simulink model "model03"  (R2018b)
settings: Solver=FixedStepAuto  StartTime=0.0  StopTime=6  FixedStep=0.001  RelTol=1e-3
values from neighbouring files (symbols this model uses):
  A_sys = [0    1 ... (first row only)    [main.m]
  B_sys = [b1 ... (first row only)    [main.m]
  C_sys = eye(2)    [main.m]
  D_sys = [0 ... (first row only)    [main.m]
  gamma = 0.1    [data.m]
  init = [1 0; -b1*k 1]^-1 * init_conds(3,:)'    [main.m]
  k = 5    [main.m]
  k1 = b^2/((V^2*sin(lambda)-b*g*cos(lambda))*m*a*c*sin(lambda))    [main.m]    (also in plotRlocus.m = 0.06)
  k2 = b*g/(V^2*sin(lambda)-b*g*cos(lambda))    [main.m]    (also in plotRlocus.m = 1.95)
settings Model: Creator=franc  LastModifiedBy=franc

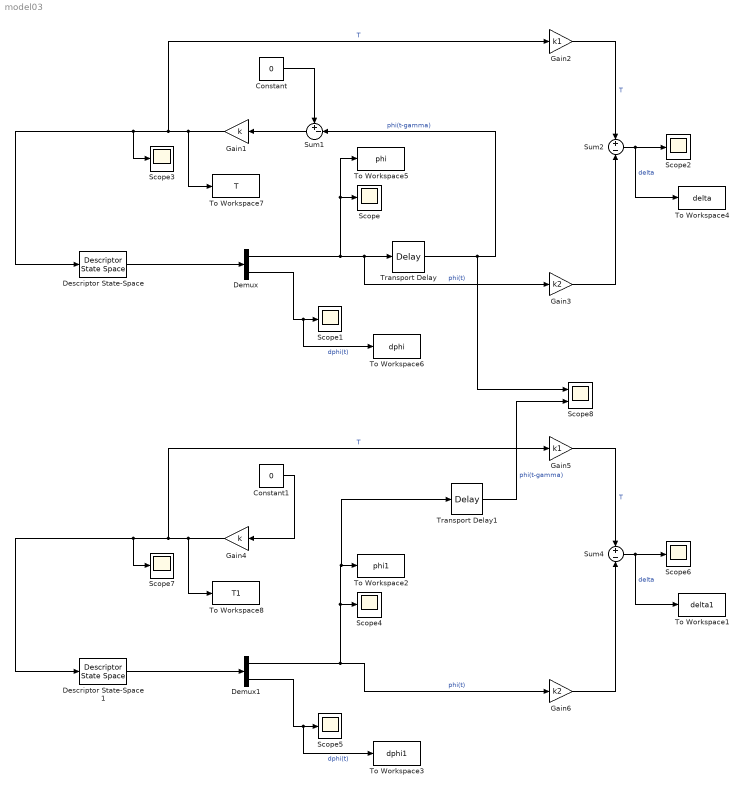
== system model03 ==
  Constant : Constant  Value=0
  Constant1 : Constant  Value=0
  Demux : Demux  Outputs=2
  Demux1 : Demux  Outputs=2
  Descriptor State-Space : DescriptorStateSpace  E=E_sys  A=A_sys  B=B_sys  C=C_sys  D=D_sys  InitialCondition=init
  Descriptor State-Space1 : DescriptorStateSpace  E=E_sys  A=A_sys  B=B_sys  C=C_sys  D=D_sys  InitialCondition=init
  Gain1 : Gain  Gain=k
  Gain2 : Gain  Gain=k1
  Gain3 : Gain  Gain=k2
  Gain4 : Gain  Gain=k
  Gain5 : Gain  Gain=k1
  Gain6 : Gain  Gain=k2
  Scope{,1..7} (8 alike) : Scope
  Scope8 : Scope  NumInputPorts=2
  Sum1 : Sum  Inputs=+-|
  Sum2 : Sum  Inputs=+|-
  Sum4 : Sum  Inputs=+|-
  To Workspace1 : ToWorkspace  VariableName=delta1  SaveFormat=Timeseries  SampleTime=-1
  To Workspace2 : ToWorkspace  VariableName=phi1  SaveFormat=Timeseries  SampleTime=-1
  To Workspace3 : ToWorkspace  VariableName=dphi1  SaveFormat=Timeseries  SampleTime=-1
  To Workspace4 : ToWorkspace  VariableName=delta  SaveFormat=Timeseries  SampleTime=-1
  To Workspace5 : ToWorkspace  VariableName=phi  SaveFormat=Timeseries  SampleTime=-1
  To Workspace6 : ToWorkspace  VariableName=dphi  SaveFormat=Timeseries  SampleTime=-1
  To Workspace7 : ToWorkspace  VariableName=T  SaveFormat=Timeseries  SampleTime=-1
  To Workspace8 : ToWorkspace  VariableName=T1  SaveFormat=Timeseries  SampleTime=-1
  Transport Delay : TransportDelay  DelayTime=gamma
  Transport Delay1 : TransportDelay  DelayTime=gamma
  wires:
  Descriptor State-Space/1 -> Demux/1
  Demux/1 -> To Workspace5/1, Scope/1, Transport Delay/1, Gain3/1  "phi(t)"
  Gain1/1 -> To Workspace7/1, Gain2/1, Scope3/1, Descriptor State-Space/1  "T"
  Demux/2 -> To Workspace6/1, Scope1/1  "dphi(t)"
  Constant/1 -> Sum1/1
  Transport Delay/1 -> Scope8/1, Sum1/2  "phi(t-gamma)"
  Sum1/1 -> Gain1/1
  Gain2/1 -> Sum2/1  "T"
  Gain3/1 -> Sum2/2
  Sum2/1 -> To Workspace4/1, Scope2/1  "delta"
  Constant1/1 -> Gain4/1
  Gain6/1 -> Sum4/2
  Demux1/2 -> To Workspace3/1, Scope5/1  "dphi(t)"
  Sum4/1 -> To Workspace1/1, Scope6/1  "delta"
  Gain4/1 -> To Workspace8/1, Gain5/1, Scope7/1, Descriptor State-Space1/1  "T"
  Gain5/1 -> Sum4/1  "T"
  Demux1/1 -> Transport Delay1/1, To Workspace2/1, Scope4/1, Gain6/1  "phi(t)"
  Descriptor State-Space1/1 -> Demux1/1
  Transport Delay1/1 -> Scope8/2  "phi(t-gamma)"
